simulink model "System_20220515"  (R2020b)
settings: Solver=ode4  StartTime=0.0  StopTime=inf  FixedStep=Ts  RelTol=1e-3  EnableMultiTasking=on
PreLoadFcn:
  | simulation_vars
PostLoadFcn:
  | simulation_vars
InitFcn:
  | simulation_vars
StartFcn:
  | simulation_vars
values from neighbouring files (symbols this model uses):
  ang_variance = 0.001*60    (= 0.06)    [simulation_vars.m]
  bus_va_seed = abs(round(1000*randn(73,1)))    [simulation_vars.m]
  bus_vm_seed = abs(round(1000*randn(73,1)))    [simulation_vars.m]
  event_time_end = event_time_start + 5/60    (= 10000.0833333)    [simulation_vars.m]
  event_time_start = 10000    [simulation_vars.m]
  line_iang0_seed = abs(round(1000*randn(104,1)))    [simulation_vars.m]
  line_iang1_seed = abs(round(1000*randn(104,1)))    [simulation_vars.m]
  line_imag0_seed = abs(round(1000*randn(104,1)))    [simulation_vars.m]
  line_imag1_seed = abs(round(1000*randn(104,1)))    [simulation_vars.m]
  mag_variance = 0.0005    [simulation_vars.m]
  spoof_lower_limit = -pi()/9    [simulation_vars.m]
  spoof_upper_limit = pi()/9    [simulation_vars.m]
  Ts = 0.001    [simulation_vars.m]
  xf_iang0_seed = abs(round(1000*randn(16,1)))    [simulation_vars.m]
  xf_iang1_seed = abs(round(1000*randn(16,1)))    [simulation_vars.m]
  xf_imag0_seed = abs(round(1000*randn(16,1)))    [simulation_vars.m]
  xf_imag1_seed = abs(round(1000*randn(16,1)))    [simulation_vars.m]
undefined symbols (not defined in the file or in its folder): en_spoofing_attack
libraries: rtlab x210, simulink x21, opal_lib x1, rtlab_phasor x1, rtio_spectracom x1
(part 3 of 4)

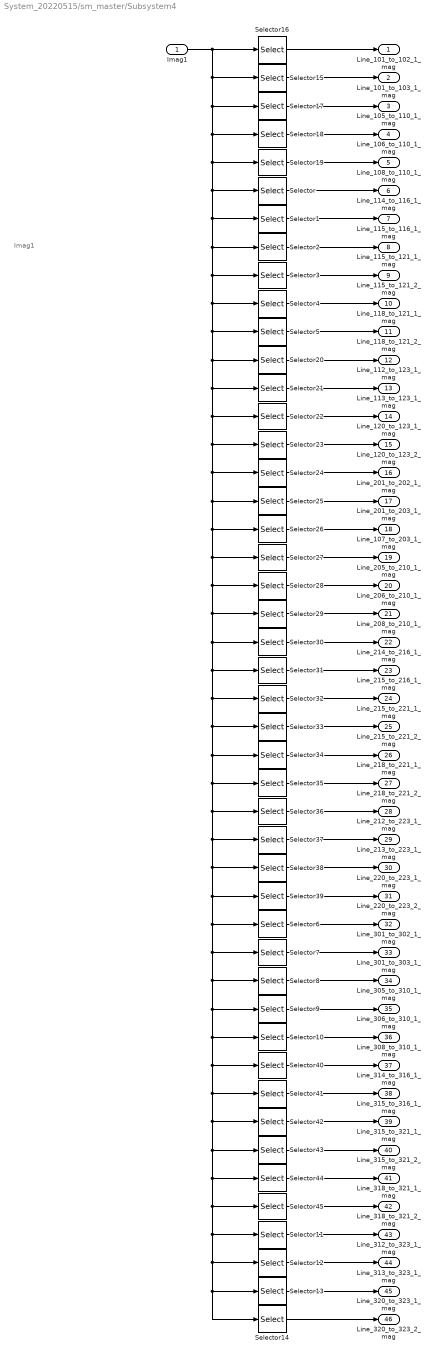
== system System_20220515/sm_master/Subsystem4 ==
  note: Imag1
  Imag1 : Inport
  Selector : Selector  InputPortWidth=104  IndexOptions=Index vector (dialog)  Indices=20  OutputSizes=1
  Selector1 : Selector  InputPortWidth=104  IndexOptions=Index vector (dialog)  Indices=21  OutputSizes=1
  Selector10 : Selector  InputPortWidth=104  IndexOptions=Index vector (dialog)  Indices=83  OutputSizes=1
  Selector11 : Selector  InputPortWidth=104  IndexOptions=Index vector (dialog)  Indices=87  OutputSizes=1
  Selector12 : Selector  InputPortWidth=104  IndexOptions=Index vector (dialog)  Indices=88  OutputSizes=1
  Selector13 : Selector  InputPortWidth=104  IndexOptions=Index vector (dialog)  Indices=102  OutputSizes=1
  Selector14 : Selector  InputPortWidth=104  IndexOptions=Index vector (dialog)  Indices=103  OutputSizes=1
  Selector15 : Selector  InputPortWidth=104  IndexOptions=Index vector (dialog)  Indices=2  OutputSizes=1
  Selector16 : Selector  InputPortWidth=104  IndexOptions=Index vector (dialog)  Indices=1  OutputSizes=1
  Selector17 : Selector  InputPortWidth=104  IndexOptions=Index vector (dialog)  Indices=8  OutputSizes=1
  Selector18 : Selector  InputPortWidth=104  IndexOptions=Index vector (dialog)  Indices=9  OutputSizes=1
  Selector19 : Selector  InputPortWidth=104  IndexOptions=Index vector (dialog)  Indices=13  OutputSizes=1
  Selector2 : Selector  InputPortWidth=104  IndexOptions=Index vector (dialog)  Indices=22  OutputSizes=1
  Selector20 : Selector  InputPortWidth=104  IndexOptions=Index vector (dialog)  Indices=17  OutputSizes=1
  Selector21 : Selector  InputPortWidth=104  IndexOptions=Index vector (dialog)  Indices=18  OutputSizes=1
  Selector22 : Selector  InputPortWidth=104  IndexOptions=Index vector (dialog)  Indices=33  OutputSizes=1
  Selector23 : Selector  InputPortWidth=104  IndexOptions=Index vector (dialog)  Indices=34  OutputSizes=1
  Selector24 : Selector  InputPortWidth=104  IndexOptions=Index vector (dialog)  Indices=38  OutputSizes=1
  Selector25 : Selector  InputPortWidth=104  IndexOptions=Index vector (dialog)  Indices=39  OutputSizes=1
  Selector26 : Selector  InputPortWidth=104  IndexOptions=Index vector (dialog)  Indices=11  OutputSizes=1
  Selector27 : Selector  InputPortWidth=104  IndexOptions=Index vector (dialog)  Indices=45  OutputSizes=1
  Selector28 : Selector  InputPortWidth=104  IndexOptions=Index vector (dialog)  Indices=46  OutputSizes=1
  Selector29 : Selector  InputPortWidth=104  IndexOptions=Index vector (dialog)  Indices=49  OutputSizes=1
  Selector3 : Selector  InputPortWidth=104  IndexOptions=Index vector (dialog)  Indices=23  OutputSizes=1
  Selector30 : Selector  InputPortWidth=104  IndexOptions=Index vector (dialog)  Indices=55  OutputSizes=1
  Selector31 : Selector  InputPortWidth=104  IndexOptions=Index vector (dialog)  Indices=56  OutputSizes=1
  Selector32 : Selector  InputPortWidth=104  IndexOptions=Index vector (dialog)  Indices=57  OutputSizes=1
  Selector33 : Selector  InputPortWidth=104  IndexOptions=Index vector (dialog)  Indices=58  OutputSizes=1
  Selector34 : Selector  InputPortWidth=104  IndexOptions=Index vector (dialog)  Indices=64  OutputSizes=1
  Selector35 : Selector  InputPortWidth=104  IndexOptions=Index vector (dialog)  Indices=65  OutputSizes=1
  Selector36 : Selector  InputPortWidth=104  IndexOptions=Index vector (dialog)  Indices=53  OutputSizes=1
  Selector37 : Selector  InputPortWidth=104  IndexOptions=Index vector (dialog)  Indices=54  OutputSizes=1
  Selector38 : Selector  InputPortWidth=104  IndexOptions=Index vector (dialog)  Indices=68  OutputSizes=1
  Selector39 : Selector  InputPortWidth=104  IndexOptions=Index vector (dialog)  Indices=69  OutputSizes=1
  Selector4 : Selector  InputPortWidth=104  IndexOptions=Index vector (dialog)  Indices=29  OutputSizes=1
  Selector40 : Selector  InputPortWidth=104  IndexOptions=Index vector (dialog)  Indices=89  OutputSizes=1
  Selector41 : Selector  InputPortWidth=104  IndexOptions=Index vector (dialog)  Indices=90  OutputSizes=1
  Selector42 : Selector  InputPortWidth=104  IndexOptions=Index vector (dialog)  Indices=91  OutputSizes=1
  Selector43 : Selector  InputPortWidth=104  IndexOptions=Index vector (dialog)  Indices=92  OutputSizes=1
  Selector44 : Selector  InputPortWidth=104  IndexOptions=Index vector (dialog)  Indices=98  OutputSizes=1
  Selector45 : Selector  InputPortWidth=104  IndexOptions=Index vector (dialog)  Indices=99  OutputSizes=1
  Selector5 : Selector  InputPortWidth=104  IndexOptions=Index vector (dialog)  Indices=30  OutputSizes=1
  Selector6 : Selector  InputPortWidth=104  IndexOptions=Index vector (dialog)  Indices=72  OutputSizes=1
  Selector7 : Selector  InputPortWidth=104  IndexOptions=Index vector (dialog)  Indices=73  OutputSizes=1
  Selector8 : Selector  InputPortWidth=104  IndexOptions=Index vector (dialog)  Indices=79  OutputSizes=1
  Selector9 : Selector  InputPortWidth=104  IndexOptions=Index vector (dialog)  Indices=80  OutputSizes=1
  Line_101_to_102_1_mag : Outport  VectorParamsAs1DForOutWhenUnconnected=off
  Line_101_to_103_1_mag : Outport  Port=2  VectorParamsAs1DForOutWhenUnconnected=off
  Line_105_to_110_1_mag : Outport  Port=3  VectorParamsAs1DForOutWhenUnconnected=off
  Line_106_to_110_1_mag : Outport  Port=4  VectorParamsAs1DForOutWhenUnconnected=off
  Line_108_to_110_1_mag : Outport  Port=5  VectorParamsAs1DForOutWhenUnconnected=off
  Line_114_to_116_1_mag : Outport  Port=6  VectorParamsAs1DForOutWhenUnconnected=off
  Line_115_to_116_1_mag : Outport  Port=7  VectorParamsAs1DForOutWhenUnconnected=off
  Line_115_to_121_1_mag : Outport  Port=8  VectorParamsAs1DForOutWhenUnconnected=off
  Line_115_to_121_2_mag : Outport  Port=9  VectorParamsAs1DForOutWhenUnconnected=off
  Line_118_to_121_1_mag : Outport  Port=10  VectorParamsAs1DForOutWhenUnconnected=off
  Line_118_to_121_2_mag : Outport  Port=11  VectorParamsAs1DForOutWhenUnconnected=off
  Line_112_to_123_1_mag : Outport  Port=12  VectorParamsAs1DForOutWhenUnconnected=off
  Line_113_to_123_1_mag : Outport  Port=13  VectorParamsAs1DForOutWhenUnconnected=off
  Line_120_to_123_1_mag : Outport  Port=14  VectorParamsAs1DForOutWhenUnconnected=off
  Line_120_to_123_2_mag : Outport  Port=15  VectorParamsAs1DForOutWhenUnconnected=off
  Line_201_to_202_1_mag : Outport  Port=16  VectorParamsAs1DForOutWhenUnconnected=off
  Line_201_to_203_1_mag : Outport  Port=17  VectorParamsAs1DForOutWhenUnconnected=off
  Line_107_to_203_1_mag : Outport  Port=18  VectorParamsAs1DForOutWhenUnconnected=off
  Line_205_to_210_1_mag : Outport  Port=19  VectorParamsAs1DForOutWhenUnconnected=off
  Line_206_to_210_1_mag : Outport  Port=20  VectorParamsAs1DForOutWhenUnconnected=off
  Line_208_to_210_1_mag : Outport  Port=21  VectorParamsAs1DForOutWhenUnconnected=off
  Line_214_to_216_1_mag : Outport  Port=22  VectorParamsAs1DForOutWhenUnconnected=off
  Line_215_to_216_1_mag : Outport  Port=23  VectorParamsAs1DForOutWhenUnconnected=off
  Line_215_to_221_1_mag : Outport  Port=24  VectorParamsAs1DForOutWhenUnconnected=off
  Line_215_to_221_2_mag : Outport  Port=25  VectorParamsAs1DForOutWhenUnconnected=off
  Line_218_to_221_1_mag : Outport  Port=26  VectorParamsAs1DForOutWhenUnconnected=off
  Line_218_to_221_2_mag : Outport  Port=27  VectorParamsAs1DForOutWhenUnconnected=off
  Line_212_to_223_1_mag : Outport  Port=28  VectorParamsAs1DForOutWhenUnconnected=off
  Line_213_to_223_1_mag : Outport  Port=29  VectorParamsAs1DForOutWhenUnconnected=off
  Line_220_to_223_1_mag : Outport  Port=30  VectorParamsAs1DForOutWhenUnconnected=off
  Line_220_to_223_2_mag : Outport  Port=31  VectorParamsAs1DForOutWhenUnconnected=off
  Line_301_to_302_1_mag : Outport  Port=32  VectorParamsAs1DForOutWhenUnconnected=off
  Line_301_to_303_1_mag : Outport  Port=33  VectorParamsAs1DForOutWhenUnconnected=off
  Line_305_to_310_1_mag : Outport  Port=34  VectorParamsAs1DForOutWhenUnconnected=off
  Line_306_to_310_1_mag : Outport  Port=35  VectorParamsAs1DForOutWhenUnconnected=off
  Line_308_to_310_1_mag : Outport  Port=36  VectorParamsAs1DForOutWhenUnconnected=off
  Line_314_to_316_1_mag : Outport  Port=37  VectorParamsAs1DForOutWhenUnconnected=off
  Line_315_to_316_1_mag : Outport  Port=38  VectorParamsAs1DForOutWhenUnconnected=off
  Line_315_to_321_1_mag : Outport  Port=39  VectorParamsAs1DForOutWhenUnconnected=off
  Line_315_to_321_2_mag : Outport  Port=40  VectorParamsAs1DForOutWhenUnconnected=off
  Line_318_to_321_1_mag : Outport  Port=41  VectorParamsAs1DForOutWhenUnconnected=off
  Line_318_to_321_2_mag : Outport  Port=42  VectorParamsAs1DForOutWhenUnconnected=off
  Line_312_to_323_1_mag : Outport  Port=43  VectorParamsAs1DForOutWhenUnconnected=off
  Line_313_to_323_1_mag : Outport  Port=44  VectorParamsAs1DForOutWhenUnconnected=off
  Line_320_to_323_1_mag : Outport  Port=45  VectorParamsAs1DForOutWhenUnconnected=off
  Line_320_to_323_2_mag : Outport  Port=46  VectorParamsAs1DForOutWhenUnconnected=off
  wires:
  Selector/1 -> Line_114_to_116_1_mag/1
  Selector1/1 -> Line_115_to_116_1_mag/1
  Selector2/1 -> Line_115_to_121_1_mag/1
  Selector3/1 -> Line_115_to_121_2_mag/1
  Selector4/1 -> Line_118_to_121_1_mag/1
  Selector5/1 -> Line_118_to_121_2_mag/1
  Selector6/1 -> Line_301_to_302_1_mag/1
  Selector7/1 -> Line_301_to_303_1_mag/1
  Selector8/1 -> Line_305_to_310_1_mag/1
  Selector9/1 -> Line_306_to_310_1_mag/1
  Selector10/1 -> Line_308_to_310_1_mag/1
  Selector11/1 -> Line_312_to_323_1_mag/1
  Selector12/1 -> Line_313_to_323_1_mag/1
  Selector13/1 -> Line_320_to_323_1_mag/1
  Selector14/1 -> Line_320_to_323_2_mag/1
  Imag1/1 -> Selector17/1, Selector18/1, Selector19/1, Selector4/1, Selector5/1, Selector20/1, Selector21/1, Selector22/1, Selector23/1, Selector24/1, Selector25/1, Selector26/1, Selector27/1, Selector28/1, Selector29/1, Selector30/1, Selector31/1, Selector32/1, Selector33/1, Selector34/1, Selector35/1, Selector36/1, Selector37/1, Selector38/1, Selector39/1, Selector8/1, Selector9/1, Selector10/1, Selector40/1, Selector41/1, Selector42/1, Selector43/1, Selector44/1, Selector45/1, Selector12/1, Selector13/1, Selector14/1, Selector11/1, Selector7/1, Selector6/1, Selector3/1, Selector2/1, Selector1/1, Selector/1, Selector15/1, Selector16/1
  Selector16/1 -> Line_101_to_102_1_mag/1
  Selector15/1 -> Line_101_to_103_1_mag/1
  Selector17/1 -> Line_105_to_110_1_mag/1
  Selector18/1 -> Line_106_to_110_1_mag/1
  Selector19/1 -> Line_108_to_110_1_mag/1
  Selector20/1 -> Line_112_to_123_1_mag/1
  Selector21/1 -> Line_113_to_123_1_mag/1
  Selector22/1 -> Line_120_to_123_1_mag/1
  Selector23/1 -> Line_120_to_123_2_mag/1
  Selector24/1 -> Line_201_to_202_1_mag/1
  Selector25/1 -> Line_201_to_203_1_mag/1
  Selector26/1 -> Line_107_to_203_1_mag/1
  Selector27/1 -> Line_205_to_210_1_mag/1
  Selector28/1 -> Line_206_to_210_1_mag/1
  Selector29/1 -> Line_208_to_210_1_mag/1
  Selector30/1 -> Line_214_to_216_1_mag/1
  Selector31/1 -> Line_215_to_216_1_mag/1
  Selector32/1 -> Line_215_to_221_1_mag/1
  Selector33/1 -> Line_215_to_221_2_mag/1
  Selector34/1 -> Line_218_to_221_1_mag/1
  Selector35/1 -> Line_218_to_221_2_mag/1
  Selector36/1 -> Line_212_to_223_1_mag/1
  Selector37/1 -> Line_213_to_223_1_mag/1
  Selector38/1 -> Line_220_to_223_1_mag/1
  Selector39/1 -> Line_220_to_223_2_mag/1
  Selector40/1 -> Line_314_to_316_1_mag/1
  Selector41/1 -> Line_315_to_316_1_mag/1
  Selector42/1 -> Line_315_to_321_1_mag/1
  Selector43/1 -> Line_315_to_321_2_mag/1
  Selector44/1 -> Line_318_to_321_1_mag/1
  Selector45/1 -> Line_318_to_321_2_mag/1

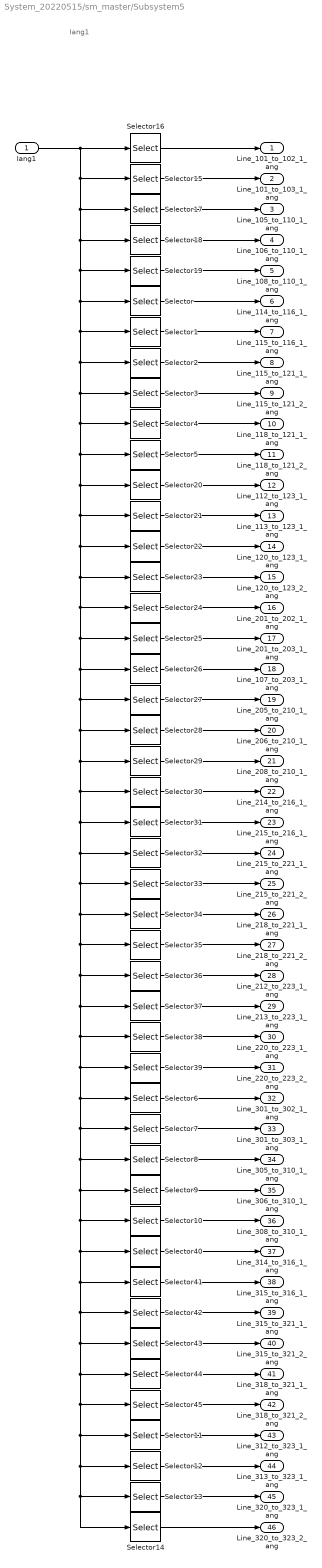
== system System_20220515/sm_master/Subsystem5 ==
  note: Iang1
  Iang1 : Inport
  Selector : Selector  InputPortWidth=104  IndexOptions=Index vector (dialog)  Indices=20  OutputSizes=1
  Selector1 : Selector  InputPortWidth=104  IndexOptions=Index vector (dialog)  Indices=21  OutputSizes=1
  Selector10 : Selector  InputPortWidth=104  IndexOptions=Index vector (dialog)  Indices=83  OutputSizes=1
  Selector11 : Selector  InputPortWidth=104  IndexOptions=Index vector (dialog)  Indices=87  OutputSizes=1
  Selector12 : Selector  InputPortWidth=104  IndexOptions=Index vector (dialog)  Indices=88  OutputSizes=1
  Selector13 : Selector  InputPortWidth=104  IndexOptions=Index vector (dialog)  Indices=102  OutputSizes=1
  Selector14 : Selector  InputPortWidth=104  IndexOptions=Index vector (dialog)  Indices=103  OutputSizes=1
  Selector15 : Selector  InputPortWidth=104  IndexOptions=Index vector (dialog)  Indices=2  OutputSizes=1
  Selector16 : Selector  InputPortWidth=104  IndexOptions=Index vector (dialog)  Indices=1  OutputSizes=1
  Selector17 : Selector  InputPortWidth=104  IndexOptions=Index vector (dialog)  Indices=8  OutputSizes=1
  Selector18 : Selector  InputPortWidth=104  IndexOptions=Index vector (dialog)  Indices=9  OutputSizes=1
  Selector19 : Selector  InputPortWidth=104  IndexOptions=Index vector (dialog)  Indices=13  OutputSizes=1
  Selector2 : Selector  InputPortWidth=104  IndexOptions=Index vector (dialog)  Indices=22  OutputSizes=1
  Selector20 : Selector  InputPortWidth=104  IndexOptions=Index vector (dialog)  Indices=17  OutputSizes=1
  Selector21 : Selector  InputPortWidth=104  IndexOptions=Index vector (dialog)  Indices=18  OutputSizes=1
  Selector22 : Selector  InputPortWidth=104  IndexOptions=Index vector (dialog)  Indices=33  OutputSizes=1
  Selector23 : Selector  InputPortWidth=104  IndexOptions=Index vector (dialog)  Indices=34  OutputSizes=1
  Selector24 : Selector  InputPortWidth=104  IndexOptions=Index vector (dialog)  Indices=38  OutputSizes=1
  Selector25 : Selector  InputPortWidth=104  IndexOptions=Index vector (dialog)  Indices=39  OutputSizes=1
  Selector26 : Selector  InputPortWidth=104  IndexOptions=Index vector (dialog)  Indices=11  OutputSizes=1
  Selector27 : Selector  InputPortWidth=104  IndexOptions=Index vector (dialog)  Indices=45  OutputSizes=1
  Selector28 : Selector  InputPortWidth=104  IndexOptions=Index vector (dialog)  Indices=46  OutputSizes=1
  Selector29 : Selector  InputPortWidth=104  IndexOptions=Index vector (dialog)  Indices=49  OutputSizes=1
  Selector3 : Selector  InputPortWidth=104  IndexOptions=Index vector (dialog)  Indices=23  OutputSizes=1
  Selector30 : Selector  InputPortWidth=104  IndexOptions=Index vector (dialog)  Indices=55  OutputSizes=1
  Selector31 : Selector  InputPortWidth=104  IndexOptions=Index vector (dialog)  Indices=56  OutputSizes=1
  Selector32 : Selector  InputPortWidth=104  IndexOptions=Index vector (dialog)  Indices=57  OutputSizes=1
  Selector33 : Selector  InputPortWidth=104  IndexOptions=Index vector (dialog)  Indices=58  OutputSizes=1
  Selector34 : Selector  InputPortWidth=104  IndexOptions=Index vector (dialog)  Indices=64  OutputSizes=1
  Selector35 : Selector  InputPortWidth=104  IndexOptions=Index vector (dialog)  Indices=65  OutputSizes=1
  Selector36 : Selector  InputPortWidth=104  IndexOptions=Index vector (dialog)  Indices=53  OutputSizes=1
  Selector37 : Selector  InputPortWidth=104  IndexOptions=Index vector (dialog)  Indices=54  OutputSizes=1
  Selector38 : Selector  InputPortWidth=104  IndexOptions=Index vector (dialog)  Indices=68  OutputSizes=1
  Selector39 : Selector  InputPortWidth=104  IndexOptions=Index vector (dialog)  Indices=69  OutputSizes=1
  Selector4 : Selector  InputPortWidth=104  IndexOptions=Index vector (dialog)  Indices=29  OutputSizes=1
  Selector40 : Selector  InputPortWidth=104  IndexOptions=Index vector (dialog)  Indices=89  OutputSizes=1
  Selector41 : Selector  InputPortWidth=104  IndexOptions=Index vector (dialog)  Indices=90  OutputSizes=1
  Selector42 : Selector  InputPortWidth=104  IndexOptions=Index vector (dialog)  Indices=91  OutputSizes=1
  Selector43 : Selector  InputPortWidth=104  IndexOptions=Index vector (dialog)  Indices=92  OutputSizes=1
  Selector44 : Selector  InputPortWidth=104  IndexOptions=Index vector (dialog)  Indices=98  OutputSizes=1
  Selector45 : Selector  InputPortWidth=104  IndexOptions=Index vector (dialog)  Indices=99  OutputSizes=1
  Selector5 : Selector  InputPortWidth=104  IndexOptions=Index vector (dialog)  Indices=30  OutputSizes=1
  Selector6 : Selector  InputPortWidth=104  IndexOptions=Index vector (dialog)  Indices=72  OutputSizes=1
  Selector7 : Selector  InputPortWidth=104  IndexOptions=Index vector (dialog)  Indices=73  OutputSizes=1
  Selector8 : Selector  InputPortWidth=104  IndexOptions=Index vector (dialog)  Indices=79  OutputSizes=1
  Selector9 : Selector  InputPortWidth=104  IndexOptions=Index vector (dialog)  Indices=80  OutputSizes=1
  Line_101_to_102_1_ang : Outport  VectorParamsAs1DForOutWhenUnconnected=off
  Line_101_to_103_1_ang : Outport  Port=2  VectorParamsAs1DForOutWhenUnconnected=off
  Line_105_to_110_1_ang : Outport  Port=3  VectorParamsAs1DForOutWhenUnconnected=off
  Line_106_to_110_1_ang : Outport  Port=4  VectorParamsAs1DForOutWhenUnconnected=off
  Line_108_to_110_1_ang : Outport  Port=5  VectorParamsAs1DForOutWhenUnconnected=off
  Line_114_to_116_1_ang : Outport  Port=6  VectorParamsAs1DForOutWhenUnconnected=off
  Line_115_to_116_1_ang : Outport  Port=7  VectorParamsAs1DForOutWhenUnconnected=off
  Line_115_to_121_1_ang : Outport  Port=8  VectorParamsAs1DForOutWhenUnconnected=off
  Line_115_to_121_2_ang : Outport  Port=9  VectorParamsAs1DForOutWhenUnconnected=off
  Line_118_to_121_1_ang : Outport  Port=10  VectorParamsAs1DForOutWhenUnconnected=off
  Line_118_to_121_2_ang : Outport  Port=11  VectorParamsAs1DForOutWhenUnconnected=off
  Line_112_to_123_1_ang : Outport  Port=12  VectorParamsAs1DForOutWhenUnconnected=off
  Line_113_to_123_1_ang : Outport  Port=13  VectorParamsAs1DForOutWhenUnconnected=off
  Line_120_to_123_1_ang : Outport  Port=14  VectorParamsAs1DForOutWhenUnconnected=off
  Line_120_to_123_2_ang : Outport  Port=15  VectorParamsAs1DForOutWhenUnconnected=off
  Line_201_to_202_1_ang : Outport  Port=16  VectorParamsAs1DForOutWhenUnconnected=off
  Line_201_to_203_1_ang : Outport  Port=17  VectorParamsAs1DForOutWhenUnconnected=off
  Line_107_to_203_1_ang : Outport  Port=18  VectorParamsAs1DForOutWhenUnconnected=off
  Line_205_to_210_1_ang : Outport  Port=19  VectorParamsAs1DForOutWhenUnconnected=off
  Line_206_to_210_1_ang : Outport  Port=20  VectorParamsAs1DForOutWhenUnconnected=off
  Line_208_to_210_1_ang : Outport  Port=21  VectorParamsAs1DForOutWhenUnconnected=off
  Line_214_to_216_1_ang : Outport  Port=22  VectorParamsAs1DForOutWhenUnconnected=off
  Line_215_to_216_1_ang : Outport  Port=23  VectorParamsAs1DForOutWhenUnconnected=off
  Line_215_to_221_1_ang : Outport  Port=24  VectorParamsAs1DForOutWhenUnconnected=off
  Line_215_to_221_2_ang : Outport  Port=25  VectorParamsAs1DForOutWhenUnconnected=off
  Line_218_to_221_1_ang : Outport  Port=26  VectorParamsAs1DForOutWhenUnconnected=off
  Line_218_to_221_2_ang : Outport  Port=27  VectorParamsAs1DForOutWhenUnconnected=off
  Line_212_to_223_1_ang : Outport  Port=28  VectorParamsAs1DForOutWhenUnconnected=off
  Line_213_to_223_1_ang : Outport  Port=29  VectorParamsAs1DForOutWhenUnconnected=off
  Line_220_to_223_1_ang : Outport  Port=30  VectorParamsAs1DForOutWhenUnconnected=off
  Line_220_to_223_2_ang : Outport  Port=31  VectorParamsAs1DForOutWhenUnconnected=off
  Line_301_to_302_1_ang : Outport  Port=32  VectorParamsAs1DForOutWhenUnconnected=off
  Line_301_to_303_1_ang : Outport  Port=33  VectorParamsAs1DForOutWhenUnconnected=off
  Line_305_to_310_1_ang : Outport  Port=34  VectorParamsAs1DForOutWhenUnconnected=off
  Line_306_to_310_1_ang : Outport  Port=35  VectorParamsAs1DForOutWhenUnconnected=off
  Line_308_to_310_1_ang : Outport  Port=36  VectorParamsAs1DForOutWhenUnconnected=off
  Line_314_to_316_1_ang : Outport  Port=37  VectorParamsAs1DForOutWhenUnconnected=off
  Line_315_to_316_1_ang : Outport  Port=38  VectorParamsAs1DForOutWhenUnconnected=off
  Line_315_to_321_1_ang : Outport  Port=39  VectorParamsAs1DForOutWhenUnconnected=off
  Line_315_to_321_2_ang : Outport  Port=40  VectorParamsAs1DForOutWhenUnconnected=off
  Line_318_to_321_1_ang : Outport  Port=41  VectorParamsAs1DForOutWhenUnconnected=off
  Line_318_to_321_2_ang : Outport  Port=42  VectorParamsAs1DForOutWhenUnconnected=off
  Line_312_to_323_1_ang : Outport  Port=43  VectorParamsAs1DForOutWhenUnconnected=off
  Line_313_to_323_1_ang : Outport  Port=44  VectorParamsAs1DForOutWhenUnconnected=off
  Line_320_to_323_1_ang : Outport  Port=45  VectorParamsAs1DForOutWhenUnconnected=off
  Line_320_to_323_2_ang : Outport  Port=46  VectorParamsAs1DForOutWhenUnconnected=off
  wires:
  Selector44/1 -> Line_318_to_321_1_ang/1
  Selector25/1 -> Line_201_to_203_1_ang/1
  Selector28/1 -> Line_206_to_210_1_ang/1
  Selector45/1 -> Line_318_to_321_2_ang/1
  Selector38/1 -> Line_220_to_223_1_ang/1
  Selector32/1 -> Line_215_to_221_1_ang/1
  Selector37/1 -> Line_213_to_223_1_ang/1
  Selector26/1 -> Line_107_to_203_1_ang/1
  Selector18/1 -> Line_106_to_110_1_ang/1
  Selector36/1 -> Line_212_to_223_1_ang/1
  Selector19/1 -> Line_108_to_110_1_ang/1
  Selector23/1 -> Line_120_to_123_2_ang/1
  Selector31/1 -> Line_215_to_216_1_ang/1
  Selector33/1 -> Line_215_to_221_2_ang/1
  Selector41/1 -> Line_315_to_316_1_ang/1
  Selector35/1 -> Line_218_to_221_2_ang/1
  Selector17/1 -> Line_105_to_110_1_ang/1
  Selector43/1 -> Line_315_to_321_2_ang/1
  Selector20/1 -> Line_112_to_123_1_ang/1
  Selector9/1 -> Line_306_to_310_1_ang/1
  Selector/1 -> Line_114_to_116_1_ang/1
  Iang1/1 -> Selector17/1, Selector18/1, Selector19/1, Selector4/1, Selector5/1, Selector20/1, Selector21/1, Selector22/1, Selector23/1, Selector24/1, Selector25/1, Selector26/1, Selector27/1, Selector28/1, Selector29/1, Selector30/1, Selector31/1, Selector32/1, Selector33/1, Selector34/1, Selector35/1, Selector36/1, Selector37/1, Selector38/1, Selector39/1, Selector8/1, Selector9/1, Selector10/1, Selector40/1, Selector41/1, Selector42/1, Selector43/1, Selector44/1, Selector45/1, Selector12/1, Selector13/1, Selector14/1, Selector11/1, Selector7/1, Selector6/1, Selector3/1, Selector2/1, Selector1/1, Selector/1, Selector15/1, Selector16/1
  Selector14/1 -> Line_320_to_323_2_ang/1
  Selector1/1 -> Line_115_to_116_1_ang/1
  Selector13/1 -> Line_320_to_323_1_ang/1
  Selector12/1 -> Line_313_to_323_1_ang/1
  Selector4/1 -> Line_118_to_121_1_ang/1
  Selector7/1 -> Line_301_to_303_1_ang/1
  Selector2/1 -> Line_115_to_121_1_ang/1
  Selector6/1 -> Line_301_to_302_1_ang/1
  Selector42/1 -> Line_315_to_321_1_ang/1
  Selector21/1 -> Line_113_to_123_1_ang/1
  Selector22/1 -> Line_120_to_123_1_ang/1
  Selector15/1 -> Line_101_to_103_1_ang/1
  Selector16/1 -> Line_101_to_102_1_ang/1
  Selector27/1 -> Line_205_to_210_1_ang/1
  Selector30/1 -> Line_214_to_216_1_ang/1
  Selector3/1 -> Line_115_to_121_2_ang/1
  Selector8/1 -> Line_305_to_310_1_ang/1
  Selector39/1 -> Line_220_to_223_2_ang/1
  Selector40/1 -> Line_314_to_316_1_ang/1
  Selector29/1 -> Line_208_to_210_1_ang/1
  Selector11/1 -> Line_312_to_323_1_ang/1
  Selector34/1 -> Line_218_to_221_1_ang/1
  Selector24/1 -> Line_201_to_202_1_ang/1
  Selector10/1 -> Line_308_to_310_1_ang/1
  Selector5/1 -> Line_118_to_121_2_ang/1

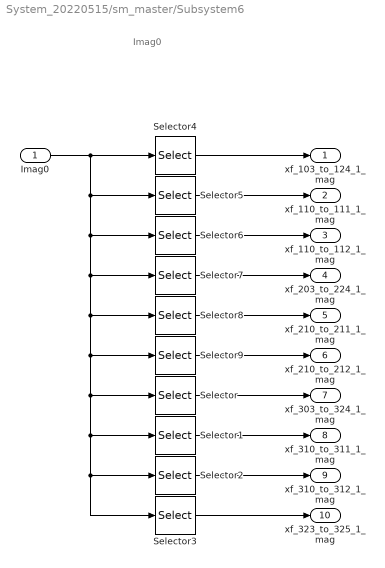
== system System_20220515/sm_master/Subsystem6 ==
  note: Imag0
  Imag0 : Inport
  Selector : Selector  InputPortWidth=16  IndexOptions=Index vector (dialog)  Indices=11  OutputSizes=1
  Selector1 : Selector  InputPortWidth=16  IndexOptions=Index vector (dialog)  Indices=14  OutputSizes=1
  Selector2 : Selector  InputPortWidth=16  IndexOptions=Index vector (dialog)  Indices=15  OutputSizes=1
  Selector3 : Selector  InputPortWidth=16  IndexOptions=Index vector (dialog)  Indices=16  OutputSizes=1
  Selector4 : Selector  InputPortWidth=16  IndexOptions=Index vector (dialog)  Indices=1  OutputSizes=1
  Selector5 : Selector  InputPortWidth=16  IndexOptions=Index vector (dialog)  Indices=4  OutputSizes=1
  Selector6 : Selector  InputPortWidth=16  IndexOptions=Index vector (dialog)  Indices=5  OutputSizes=1
  Selector7 : Selector  InputPortWidth=16  IndexOptions=Index vector (dialog)  Indices=6  OutputSizes=1
  Selector8 : Selector  InputPortWidth=16  IndexOptions=Index vector (dialog)  Indices=9  OutputSizes=1
  Selector9 : Selector  InputPortWidth=16  IndexOptions=Index vector (dialog)  Indices=10  OutputSizes=1
  xf_103_to_124_1_mag : Outport  VectorParamsAs1DForOutWhenUnconnected=off
  xf_110_to_111_1_mag : Outport  Port=2  VectorParamsAs1DForOutWhenUnconnected=off
  xf_110_to_112_1_mag : Outport  Port=3  VectorParamsAs1DForOutWhenUnconnected=off
  xf_203_to_224_1_mag : Outport  Port=4  VectorParamsAs1DForOutWhenUnconnected=off
  xf_210_to_211_1_mag : Outport  Port=5  VectorParamsAs1DForOutWhenUnconnected=off
  xf_210_to_212_1_mag : Outport  Port=6  VectorParamsAs1DForOutWhenUnconnected=off
  xf_303_to_324_1_mag : Outport  Port=7  VectorParamsAs1DForOutWhenUnconnected=off
  xf_310_to_311_1_mag : Outport  Port=8  VectorParamsAs1DForOutWhenUnconnected=off
  xf_310_to_312_1_mag : Outport  Port=9  VectorParamsAs1DForOutWhenUnconnected=off
  xf_323_to_325_1_mag : Outport  Port=10  VectorParamsAs1DForOutWhenUnconnected=off
  wires:
  Selector/1 -> xf_303_to_324_1_mag/1
  Selector1/1 -> xf_310_to_311_1_mag/1
  Selector2/1 -> xf_310_to_312_1_mag/1
  Imag0/1 -> Selector4/1, Selector5/1, Selector6/1, Selector7/1, Selector3/1, Selector2/1, Selector1/1, Selector/1, Selector9/1, Selector8/1
  Selector3/1 -> xf_323_to_325_1_mag/1
  Selector4/1 -> xf_103_to_124_1_mag/1
  Selector5/1 -> xf_110_to_111_1_mag/1
  Selector6/1 -> xf_110_to_112_1_mag/1
  Selector7/1 -> xf_203_to_224_1_mag/1
  Selector8/1 -> xf_210_to_211_1_mag/1
  Selector9/1 -> xf_210_to_212_1_mag/1

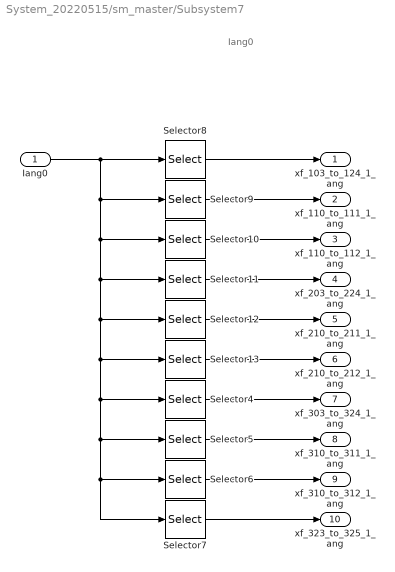
== system System_20220515/sm_master/Subsystem7 ==
  note: Iang0
  Iang0 : Inport
  Selector10 : Selector  InputPortWidth=16  IndexOptions=Index vector (dialog)  Indices=5  OutputSizes=1
  Selector11 : Selector  InputPortWidth=16  IndexOptions=Index vector (dialog)  Indices=6  OutputSizes=1
  Selector12 : Selector  InputPortWidth=16  IndexOptions=Index vector (dialog)  Indices=9  OutputSizes=1
  Selector13 : Selector  InputPortWidth=16  IndexOptions=Index vector (dialog)  Indices=10  OutputSizes=1
  Selector4 : Selector  InputPortWidth=16  IndexOptions=Index vector (dialog)  Indices=11  OutputSizes=1
  Selector5 : Selector  InputPortWidth=16  IndexOptions=Index vector (dialog)  Indices=14  OutputSizes=1
  Selector6 : Selector  InputPortWidth=16  IndexOptions=Index vector (dialog)  Indices=15  OutputSizes=1
  Selector7 : Selector  InputPortWidth=16  IndexOptions=Index vector (dialog)  Indices=16  OutputSizes=1
  Selector8 : Selector  InputPortWidth=16  IndexOptions=Index vector (dialog)  Indices=1  OutputSizes=1
  Selector9 : Selector  InputPortWidth=16  IndexOptions=Index vector (dialog)  Indices=4  OutputSizes=1
  xf_103_to_124_1_ang : Outport  VectorParamsAs1DForOutWhenUnconnected=off
  xf_110_to_111_1_ang : Outport  Port=2  VectorParamsAs1DForOutWhenUnconnected=off
  xf_110_to_112_1_ang : Outport  Port=3  VectorParamsAs1DForOutWhenUnconnected=off
  xf_203_to_224_1_ang : Outport  Port=4  VectorParamsAs1DForOutWhenUnconnected=off
  xf_210_to_211_1_ang : Outport  Port=5  VectorParamsAs1DForOutWhenUnconnected=off
  xf_210_to_212_1_ang : Outport  Port=6  VectorParamsAs1DForOutWhenUnconnected=off
  xf_303_to_324_1_ang : Outport  Port=7  VectorParamsAs1DForOutWhenUnconnected=off
  xf_310_to_311_1_ang : Outport  Port=8  VectorParamsAs1DForOutWhenUnconnected=off
  xf_310_to_312_1_ang : Outport  Port=9  VectorParamsAs1DForOutWhenUnconnected=off
  xf_323_to_325_1_ang : Outport  Port=10  VectorParamsAs1DForOutWhenUnconnected=off
  wires:
  Selector13/1 -> xf_210_to_212_1_ang/1
  Selector10/1 -> xf_110_to_112_1_ang/1
  Selector12/1 -> xf_210_to_211_1_ang/1
  Selector11/1 -> xf_203_to_224_1_ang/1
  Selector4/1 -> xf_303_to_324_1_ang/1
  Iang0/1 -> Selector8/1, Selector9/1, Selector10/1, Selector11/1, Selector7/1, Selector6/1, Selector5/1, Selector4/1, Selector13/1, Selector12/1
  Selector9/1 -> xf_110_to_111_1_ang/1
  Selector7/1 -> xf_323_to_325_1_ang/1
  Selector6/1 -> xf_310_to_312_1_ang/1
  Selector5/1 -> xf_310_to_311_1_ang/1
  Selector8/1 -> xf_103_to_124_1_ang/1

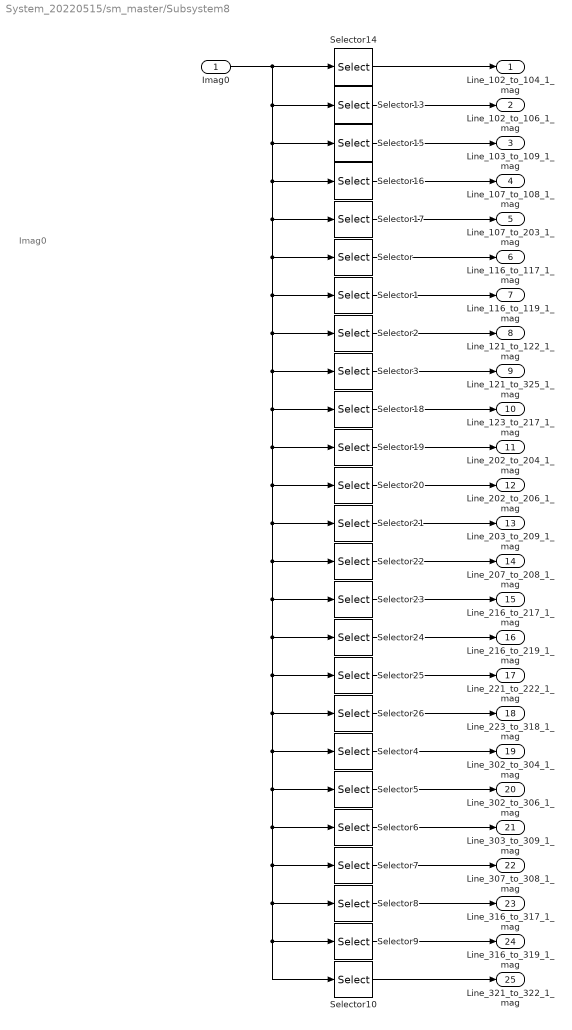
== system System_20220515/sm_master/Subsystem8 ==
  note: Imag0
  Imag0 : Inport
  Selector : Selector  InputPortWidth=104  IndexOptions=Index vector (dialog)  Indices=25  OutputSizes=1
  Selector1 : Selector  InputPortWidth=104  IndexOptions=Index vector (dialog)  Indices=26  OutputSizes=1
  Selector10 : Selector  InputPortWidth=104  IndexOptions=Index vector (dialog)  Indices=104  OutputSizes=1
  Selector13 : Selector  InputPortWidth=104  IndexOptions=Index vector (dialog)  Indices=5  OutputSizes=1
  Selector14 : Selector  InputPortWidth=104  IndexOptions=Index vector (dialog)  Indices=4  OutputSizes=1
  Selector15 : Selector  InputPortWidth=104  IndexOptions=Index vector (dialog)  Indices=6  OutputSizes=1
  Selector16 : Selector  InputPortWidth=104  IndexOptions=Index vector (dialog)  Indices=10  OutputSizes=1
  Selector17 : Selector  InputPortWidth=104  IndexOptions=Index vector (dialog)  Indices=11  OutputSizes=1
  Selector18 : Selector  InputPortWidth=104  IndexOptions=Index vector (dialog)  Indices=37  OutputSizes=1
  Selector19 : Selector  InputPortWidth=104  IndexOptions=Index vector (dialog)  Indices=41  OutputSizes=1
  Selector2 : Selector  InputPortWidth=104  IndexOptions=Index vector (dialog)  Indices=35  OutputSizes=1
  Selector20 : Selector  InputPortWidth=104  IndexOptions=Index vector (dialog)  Indices=42  OutputSizes=1
  Selector21 : Selector  InputPortWidth=104  IndexOptions=Index vector (dialog)  Indices=43  OutputSizes=1
  Selector22 : Selector  InputPortWidth=104  IndexOptions=Index vector (dialog)  Indices=47  OutputSizes=1
  Selector23 : Selector  InputPortWidth=104  IndexOptions=Index vector (dialog)  Indices=60  OutputSizes=1
  Selector24 : Selector  InputPortWidth=104  IndexOptions=Index vector (dialog)  Indices=61  OutputSizes=1
  Selector25 : Selector  InputPortWidth=104  IndexOptions=Index vector (dialog)  Indices=70  OutputSizes=1
  Selector26 : Selector  InputPortWidth=104  IndexOptions=Index vector (dialog)  Indices=71  OutputSizes=1
  Selector3 : Selector  InputPortWidth=104  IndexOptions=Index vector (dialog)  Indices=36  OutputSizes=1
  Selector4 : Selector  InputPortWidth=104  IndexOptions=Index vector (dialog)  Indices=75  OutputSizes=1
  Selector5 : Selector  InputPortWidth=104  IndexOptions=Index vector (dialog)  Indices=76  OutputSizes=1
  Selector6 : Selector  InputPortWidth=104  IndexOptions=Index vector (dialog)  Indices=77  OutputSizes=1
  Selector7 : Selector  InputPortWidth=104  IndexOptions=Index vector (dialog)  Indices=81  OutputSizes=1
  Selector8 : Selector  InputPortWidth=104  IndexOptions=Index vector (dialog)  Indices=94  OutputSizes=1
  Selector9 : Selector  InputPortWidth=104  IndexOptions=Index vector (dialog)  Indices=95  OutputSizes=1
  Line_102_to_104_1_mag : Outport  VectorParamsAs1DForOutWhenUnconnected=off
  Line_102_to_106_1_mag : Outport  Port=2  VectorParamsAs1DForOutWhenUnconnected=off
  Line_103_to_109_1_mag : Outport  Port=3  VectorParamsAs1DForOutWhenUnconnected=off
  Line_107_to_108_1_mag : Outport  Port=4  VectorParamsAs1DForOutWhenUnconnected=off
  Line_107_to_203_1_mag : Outport  Port=5  VectorParamsAs1DForOutWhenUnconnected=off
  Line_116_to_117_1_mag : Outport  Port=6  VectorParamsAs1DForOutWhenUnconnected=off
  Line_116_to_119_1_mag : Outport  Port=7  VectorParamsAs1DForOutWhenUnconnected=off
  Line_121_to_122_1_mag : Outport  Port=8  VectorParamsAs1DForOutWhenUnconnected=off
  Line_121_to_325_1_mag : Outport  Port=9  VectorParamsAs1DForOutWhenUnconnected=off
  Line_123_to_217_1_mag : Outport  Port=10  VectorParamsAs1DForOutWhenUnconnected=off
  Line_202_to_204_1_mag : Outport  Port=11  VectorParamsAs1DForOutWhenUnconnected=off
  Line_202_to_206_1_mag : Outport  Port=12  VectorParamsAs1DForOutWhenUnconnected=off
  Line_203_to_209_1_mag : Outport  Port=13  VectorParamsAs1DForOutWhenUnconnected=off
  Line_207_to_208_1_mag : Outport  Port=14  VectorParamsAs1DForOutWhenUnconnected=off
  Line_216_to_217_1_mag : Outport  Port=15  VectorParamsAs1DForOutWhenUnconnected=off
  Line_216_to_219_1_mag : Outport  Port=16  VectorParamsAs1DForOutWhenUnconnected=off
  Line_221_to_222_1_mag : Outport  Port=17  VectorParamsAs1DForOutWhenUnconnected=off
  Line_223_to_318_1_mag : Outport  Port=18  VectorParamsAs1DForOutWhenUnconnected=off
  Line_302_to_304_1_mag : Outport  Port=19  VectorParamsAs1DForOutWhenUnconnected=off
  Line_302_to_306_1_mag : Outport  Port=20  VectorParamsAs1DForOutWhenUnconnected=off
  Line_303_to_309_1_mag : Outport  Port=21  VectorParamsAs1DForOutWhenUnconnected=off
  Line_307_to_308_1_mag : Outport  Port=22  VectorParamsAs1DForOutWhenUnconnected=off
  Line_316_to_317_1_mag : Outport  Port=23  VectorParamsAs1DForOutWhenUnconnected=off
  Line_316_to_319_1_mag : Outport  Port=24  VectorParamsAs1DForOutWhenUnconnected=off
  Line_321_to_322_1_mag : Outport  Port=25  VectorParamsAs1DForOutWhenUnconnected=off
  wires:
  Selector/1 -> Line_116_to_117_1_mag/1
  Selector1/1 -> Line_116_to_119_1_mag/1
  Selector2/1 -> Line_121_to_122_1_mag/1
  Selector3/1 -> Line_121_to_325_1_mag/1
  Selector4/1 -> Line_302_to_304_1_mag/1
  Selector5/1 -> Line_302_to_306_1_mag/1
  Selector6/1 -> Line_303_to_309_1_mag/1
  Selector7/1 -> Line_307_to_308_1_mag/1
  Selector13/1 -> Line_102_to_106_1_mag/1
  Selector14/1 -> Line_102_to_104_1_mag/1
  Selector15/1 -> Line_103_to_109_1_mag/1
  Selector16/1 -> Line_107_to_108_1_mag/1
  Selector17/1 -> Line_107_to_203_1_mag/1
  Imag0/1 -> Selector3/1, Selector18/1, Selector19/1, Selector20/1, Selector21/1, Selector22/1, Selector23/1, Selector24/1, Selector26/1, Selector4/1, Selector5/1, Selector6/1, Selector10/1, Selector9/1, Selector8/1, Selector7/1, Selector25/1, Selector2/1, Selector1/1, Selector/1, Selector17/1, Selector16/1, Selector15/1, Selector13/1, Selector14/1
  Selector18/1 -> Line_123_to_217_1_mag/1
  Selector19/1 -> Line_202_to_204_1_mag/1
  Selector20/1 -> Line_202_to_206_1_mag/1
  Selector21/1 -> Line_203_to_209_1_mag/1
  Selector22/1 -> Line_207_to_208_1_mag/1
  Selector23/1 -> Line_216_to_217_1_mag/1
  Selector24/1 -> Line_216_to_219_1_mag/1
  Selector25/1 -> Line_221_to_222_1_mag/1
  Selector26/1 -> Line_223_to_318_1_mag/1
  Selector8/1 -> Line_316_to_317_1_mag/1
  Selector9/1 -> Line_316_to_319_1_mag/1
  Selector10/1 -> Line_321_to_322_1_mag/1

== system System_20220515/sm_master/Subsystem9 ==
  note: Imag1
  Imag1 : Inport
  Terminator : Terminator
  wires:
  Imag1/1 -> Terminator/1

== system System_20220515/sm_master/Timestamp selector ==
  ts_in : Inport
  Demux : Demux  Outputs=8
  Terminator{,1..4} (5 alike) : Terminator
  clock_epoch : rtlab/OpOutput  identifier_use=clock_epoch  identifier_hide=clock_epoch  nb_parents_identifier=0
      settings: SourceProductName=RT-LAB
  clock_ns : rtlab/OpOutput  identifier_use=clock_ns  identifier_hide=clock_ns  nb_parents_identifier=0
      settings: SourceProductName=RT-LAB
  clock_sync : rtlab/OpOutput  identifier_use=clock_sync  identifier_hide=clock_sync  nb_parents_identifier=0
      settings: SourceProductName=RT-LAB
  wires:
  Demux/7 -> clock_epoch/1
  Demux/6 -> clock_ns/1
  Demux/8 -> clock_sync/1
  Demux/1 -> Terminator/1
  Demux/2 -> Terminator1/1
  Demux/3 -> Terminator2/1
  Demux/4 -> Terminator3/1
  Demux/5 -> Terminator4/1
  ts_in/1 -> Demux/1

== system System_20220515/sm_master/bus_va_noise ==
  In1 : Inport
  Add1 : Sum
  MATLAB Function : MATLAB Function  TreatAsAtomicUnit=on
  Random Number : RandomNumber  Variance=ang_variance  Seed=bus_va_seed  SampleTime=Ts
  y : Outport
  wires:
  In1/1 -> Add1/1
  Random Number/1 -> Add1/2
  MATLAB Function/1(y) -> y/1
  Add1/1 -> MATLAB Function/1(u)

== system System_20220515/sm_master/bus_vm_noise ==
  In1 : Inport
  Add1 : Sum
  Random Number : RandomNumber  Variance=mag_variance  Seed=bus_vm_seed  SampleTime=Ts
  Bus_Vm : Outport
  wires:
  In1/1 -> Add1/1
  Random Number/1 -> Add1/2
  Add1/1 -> Bus_Vm/1

== system System_20220515/sm_master/line_iang0_noise ==
  In1 : Inport
  Add1 : Sum
  MATLAB Function : MATLAB Function  TreatAsAtomicUnit=on
  Random Number : RandomNumber  Variance=ang_variance  Seed=line_iang0_seed  SampleTime=Ts
  y : Outport
  wires:
  In1/1 -> Add1/1
  Random Number/1 -> Add1/2
  Add1/1 -> MATLAB Function/1(u)
  MATLAB Function/1(y) -> y/1

== system System_20220515/sm_master/line_iang1_noise ==
  In1 : Inport
  Add1 : Sum
  MATLAB Function : MATLAB Function  TreatAsAtomicUnit=on
  Random Number : RandomNumber  Variance=ang_variance  Seed=line_iang1_seed  SampleTime=Ts
  y : Outport
  wires:
  In1/1 -> Add1/1
  Random Number/1 -> Add1/2
  MATLAB Function/1(y) -> y/1
  Add1/1 -> MATLAB Function/1(u)

== system System_20220515/sm_master/line_imag0_noise ==
  In1 : Inport
  Add1 : Sum
  Random Number : RandomNumber  Variance=mag_variance  Seed=line_imag0_seed  SampleTime=Ts
  Out1 : Outport
  wires:
  In1/1 -> Add1/1
  Random Number/1 -> Add1/2
  Add1/1 -> Out1/1

== system System_20220515/sm_master/line_imag1_noise ==
  In1 : Inport
  Add1 : Sum
  Random Number : RandomNumber  Variance=mag_variance  Seed=line_imag1_seed  SampleTime=Ts
  Out1 : Outport
  wires:
  In1/1 -> Add1/1
  Random Number/1 -> Add1/2
  Add1/1 -> Out1/1

== system System_20220515/sm_master/xf_iang0_noise ==
  In1 : Inport
  Add1 : Sum
  MATLAB Function : MATLAB Function  TreatAsAtomicUnit=on
  Random Number : RandomNumber  Variance=ang_variance  Seed=xf_iang0_seed  SampleTime=Ts
  y : Outport
  wires:
  In1/1 -> Add1/1
  Random Number/1 -> Add1/2
  MATLAB Function/1(y) -> y/1
  Add1/1 -> MATLAB Function/1(u)

== system System_20220515/sm_master/xf_iang1_noise ==
  In1 : Inport
  Add1 : Sum
  MATLAB Function : MATLAB Function  TreatAsAtomicUnit=on
  Random Number : RandomNumber  Variance=ang_variance  Seed=xf_iang1_seed  SampleTime=Ts
  y : Outport
  wires:
  In1/1 -> Add1/1
  Random Number/1 -> Add1/2
  Add1/1 -> MATLAB Function/1(u)
  MATLAB Function/1(y) -> y/1

== system System_20220515/sm_master/xf_imag0_noise ==
  In1 : Inport
  Add1 : Sum
  Random Number : RandomNumber  Variance=mag_variance  Seed=xf_imag0_seed  SampleTime=Ts
  Out1 : Outport
  wires:
  In1/1 -> Add1/1
  Random Number/1 -> Add1/2
  Add1/1 -> Out1/1

== system System_20220515/sm_master/xf_imag1_noise ==
  In1 : Inport
  Add1 : Sum
  Random Number : RandomNumber  Variance=mag_variance  Seed=xf_imag1_seed  SampleTime=Ts
  Out1 : Outport
  wires:
  In1/1 -> Add1/1
  Random Number/1 -> Add1/2
  Add1/1 -> Out1/1

== system System_20220515/sm_master/PMU102_signals/Spoofing attack ==
  note: Modify demux and mux to fit input size.
      | Only modifies the angle measurements.
  Input : Inport
  Add : Sum
  Constant : Constant  Value=en_spoofing_attack.pmu_102
  Demux : Demux  Outputs=8
  Demux1 : Demux
  Multiply : Product
  Mux : Mux  Inputs=8
  Mux1 : Mux
  Ramp : simulink/Sources/Ramp  slope=1*pi()/180  start=spoof_st.pmu_102  InitialOutput=0
  Saturation : Saturate  UpperLimit=spoof_upper_limit  LowerLimit=spoof_lower_limit
  Output : Outport  VectorParamsAs1DForOutWhenUnconnected=off
  wires:
  Multiply/1 -> Add/1
  Saturation/1 -> Multiply/1
  Constant/1 -> Multiply/2
  Ramp/1 -> Saturation/1
  Input/1 -> Demux/1
  Mux/1 -> Output/1
  Demux/1 -> Mux/1
  Demux/3 -> Mux/3
  Demux/5 -> Mux/5
  Demux/7 -> Mux/7
  Demux/8 -> Mux1/4
  Demux/6 -> Mux1/3
  Demux/4 -> Mux1/2
  Demux/2 -> Mux1/1
  Mux1/1 -> Add/2
  Add/1 -> Demux1/1
  Demux1/1 -> Mux/2
  Demux1/2 -> Mux/4
  Demux1/3 -> Mux/6
  Demux1/4 -> Mux/8

== system System_20220515/sm_master/PMU103_signals/Spoofing attack ==
  note: Modify demux and mux to fit input size.
      | Only modifies the angle measurements.
  Input : Inport
  Add : Sum
  Constant : Constant  Value=en_spoofing_attack.pmu_103
  Demux : Demux  Outputs=8
  Demux1 : Demux
  Multiply : Product
  Mux : Mux  Inputs=8
  Mux1 : Mux
  Ramp : simulink/Sources/Ramp  slope=1*pi()/180  start=spoof_st.pmu_103  InitialOutput=0
  Saturation : Saturate  UpperLimit=spoof_upper_limit  LowerLimit=spoof_lower_limit
  Output : Outport  VectorParamsAs1DForOutWhenUnconnected=off
  wires:
  Multiply/1 -> Add/1
  Saturation/1 -> Multiply/1
  Constant/1 -> Multiply/2
  Ramp/1 -> Saturation/1
  Input/1 -> Demux/1
  Mux/1 -> Output/1
  Demux/1 -> Mux/1
  Demux/3 -> Mux/3
  Demux/5 -> Mux/5
  Demux/7 -> Mux/7
  Demux/8 -> Mux1/4
  Demux/6 -> Mux1/3
  Demux/4 -> Mux1/2
  Demux/2 -> Mux1/1
  Mux1/1 -> Add/2
  Add/1 -> Demux1/1
  Demux1/1 -> Mux/2
  Demux1/2 -> Mux/4
  Demux1/3 -> Mux/6
  Demux1/4 -> Mux/8

== system System_20220515/sm_master/PMU107_signals/Spoofing attack ==
  note: Modify demux and mux to fit input size.
      | Only modifies the angle measurements.
  Input : Inport
  Add : Sum
  Constant : Constant  Value=en_spoofing_attack.pmu_107
  Demux : Demux  Outputs=6
  Demux1 : Demux  Outputs=3
  Multiply : Product
  Mux : Mux  Inputs=6
  Mux1 : Mux  Inputs=3
  Ramp : simulink/Sources/Ramp  slope=1*pi()/180  start=spoof_st.pmu_107  InitialOutput=0
  Saturation : Saturate  UpperLimit=spoof_upper_limit  LowerLimit=spoof_lower_limit
  Output : Outport  VectorParamsAs1DForOutWhenUnconnected=off
  wires:
  Multiply/1 -> Add/1
  Saturation/1 -> Multiply/1
  Constant/1 -> Multiply/2
  Ramp/1 -> Saturation/1
  Input/1 -> Demux/1
  Mux/1 -> Output/1
  Demux/1 -> Mux/1
  Demux/3 -> Mux/3
  Demux/5 -> Mux/5
  Demux/6 -> Mux1/3
  Demux/4 -> Mux1/2
  Demux/2 -> Mux1/1
  Mux1/1 -> Add/2
  Add/1 -> Demux1/1
  Demux1/1 -> Mux/2
  Demux1/2 -> Mux/4
  Demux1/3 -> Mux/6

== system System_20220515/sm_master/PMU110_signals/Spoofing attack ==
  note: Modify demux and mux to fit input size.
      | Only modifies the angle measurements.
  Input : Inport
  Add : Sum
  Constant : Constant  Value=en_spoofing_attack.pmu_110
  Demux : Demux  Outputs=12
  Demux1 : Demux  Outputs=6
  Multiply : Product
  Mux : Mux  Inputs=12
  Mux1 : Mux  Inputs=6
  Ramp : simulink/Sources/Ramp  slope=1*pi()/180  start=spoof_st.pmu_110  InitialOutput=0
  Saturation : Saturate  UpperLimit=spoof_upper_limit  LowerLimit=spoof_lower_limit
  Output : Outport  VectorParamsAs1DForOutWhenUnconnected=off
  wires:
  Multiply/1 -> Add/1
  Saturation/1 -> Multiply/1
  Constant/1 -> Multiply/2
  Ramp/1 -> Saturation/1
  Input/1 -> Demux/1
  Mux/1 -> Output/1
  Demux/1 -> Mux/1
  Demux/3 -> Mux/3
  Demux/5 -> Mux/5
  Demux/7 -> Mux/7
  Demux/9 -> Mux/9
  Demux/10 -> Mux1/5
  Demux/8 -> Mux1/4
  Demux/6 -> Mux1/3
  Demux/4 -> Mux1/2
  Demux/2 -> Mux1/1
  Mux1/1 -> Add/2
  Add/1 -> Demux1/1
  Demux1/1 -> Mux/2
  Demux1/2 -> Mux/4
  Demux1/3 -> Mux/6
  Demux1/4 -> Mux/8
  Demux1/5 -> Mux/10
  Demux/11 -> Mux/11
  Demux/12 -> Mux1/6
  Demux1/6 -> Mux/12

== system System_20220515/sm_master/PMU116_signals/Spoofing attack ==
  note: Modify demux and mux to fit input size.
      | Only modifies the angle measurements.
  Input : Inport
  Add : Sum
  Constant : Constant  Value=en_spoofing_attack.pmu_116
  Demux : Demux  Outputs=10
  Demux1 : Demux  Outputs=5
  Multiply : Product
  Mux : Mux  Inputs=10
  Mux1 : Mux  Inputs=5
  Ramp : simulink/Sources/Ramp  slope=1*pi()/180  start=spoof_st.pmu_116  InitialOutput=0
  Saturation : Saturate  UpperLimit=spoof_upper_limit  LowerLimit=spoof_lower_limit
  Output : Outport  VectorParamsAs1DForOutWhenUnconnected=off
  wires:
  Multiply/1 -> Add/1
  Saturation/1 -> Multiply/1
  Constant/1 -> Multiply/2
  Ramp/1 -> Saturation/1
  Input/1 -> Demux/1
  Mux/1 -> Output/1
  Demux/1 -> Mux/1
  Demux/3 -> Mux/3
  Demux/5 -> Mux/5
  Demux/7 -> Mux/7
  Demux/9 -> Mux/9
  Demux/10 -> Mux1/5
  Demux/8 -> Mux1/4
  Demux/6 -> Mux1/3
  Demux/4 -> Mux1/2
  Demux/2 -> Mux1/1
  Mux1/1 -> Add/2
  Add/1 -> Demux1/1
  Demux1/1 -> Mux/2
  Demux1/2 -> Mux/4
  Demux1/3 -> Mux/6
  Demux1/4 -> Mux/8
  Demux1/5 -> Mux/10

== system System_20220515/sm_master/PMU121_signals/Spoofing attack ==
  note: Modify demux and mux to fit input size.
      | Only modifies the angle measurements.
  Input : Inport
  Add : Sum
  Constant : Constant  Value=en_spoofing_attack.pmu_121
  Demux : Demux  Outputs=14
  Demux1 : Demux  Outputs=7
  Multiply : Product
  Mux : Mux  Inputs=14
  Mux1 : Mux  Inputs=7
  Ramp : simulink/Sources/Ramp  slope=1*pi()/180  start=spoof_st.pmu_121  InitialOutput=0
  Saturation : Saturate  UpperLimit=spoof_upper_limit  LowerLimit=spoof_lower_limit
  Output : Outport  VectorParamsAs1DForOutWhenUnconnected=off
  wires:
  Multiply/1 -> Add/1
  Saturation/1 -> Multiply/1
  Constant/1 -> Multiply/2
  Ramp/1 -> Saturation/1
  Input/1 -> Demux/1
  Mux/1 -> Output/1
  Demux/1 -> Mux/1
  Demux/3 -> Mux/3
  Demux/5 -> Mux/5
  Demux/7 -> Mux/7
  Demux/9 -> Mux/9
  Demux/10 -> Mux1/5
  Demux/8 -> Mux1/4
  Demux/6 -> Mux1/3
  Demux/4 -> Mux1/2
  Demux/2 -> Mux1/1
  Mux1/1 -> Add/2
  Add/1 -> Demux1/1
  Demux1/1 -> Mux/2
  Demux1/2 -> Mux/4
  Demux1/3 -> Mux/6
  Demux1/4 -> Mux/8
  Demux1/5 -> Mux/10
  Demux/11 -> Mux/11
  Demux/13 -> Mux/13
  Demux1/6 -> Mux/12
  Demux1/7 -> Mux/14
  Demux/12 -> Mux1/6
  Demux/14 -> Mux1/7

== system System_20220515/sm_master/PMU123_signals/Spoofing attack ==
  note: Modify demux and mux to fit input size.
      | Only modifies the angle measurements.
  Input : Inport
  Add : Sum
  Constant : Constant  Value=en_spoofing_attack.pmu_123
  Demux : Demux  Outputs=12
  Demux1 : Demux  Outputs=6
  Multiply : Product
  Mux : Mux  Inputs=12
  Mux1 : Mux  Inputs=6
  Ramp : simulink/Sources/Ramp  slope=1*pi()/180  start=spoof_st.pmu_123  InitialOutput=0
  Saturation : Saturate  UpperLimit=spoof_upper_limit  LowerLimit=spoof_lower_limit
  Output : Outport  VectorParamsAs1DForOutWhenUnconnected=off
  wires:
  Multiply/1 -> Add/1
  Saturation/1 -> Multiply/1
  Constant/1 -> Multiply/2
  Ramp/1 -> Saturation/1
  Input/1 -> Demux/1
  Mux/1 -> Output/1
  Demux/1 -> Mux/1
  Demux/3 -> Mux/3
  Demux/5 -> Mux/5
  Demux/7 -> Mux/7
  Demux/9 -> Mux/9
  Demux/10 -> Mux1/5
  Demux/8 -> Mux1/4
  Demux/6 -> Mux1/3
  Demux/4 -> Mux1/2
  Demux/2 -> Mux1/1
  Mux1/1 -> Add/2
  Add/1 -> Demux1/1
  Demux1/1 -> Mux/2
  Demux1/2 -> Mux/4
  Demux1/3 -> Mux/6
  Demux1/4 -> Mux/8
  Demux1/5 -> Mux/10
  Demux/11 -> Mux/11
  Demux/12 -> Mux1/6
  Demux1/6 -> Mux/12

== system System_20220515/sm_master/PMU202_signals/Spoofing attack ==
  note: Modify demux and mux to fit input size.
      | Only modifies the angle measurements.
  Input : Inport
  Add : Sum
  Constant : Constant  Value=en_spoofing_attack.pmu_202
  Demux : Demux  Outputs=8
  Demux1 : Demux
  Multiply : Product
  Mux : Mux  Inputs=8
  Mux1 : Mux
  Ramp : simulink/Sources/Ramp  slope=1*pi()/180  start=spoof_st.pmu_202  InitialOutput=0
  Saturation : Saturate  UpperLimit=spoof_upper_limit  LowerLimit=spoof_lower_limit
  Output : Outport  VectorParamsAs1DForOutWhenUnconnected=off
  wires:
  Multiply/1 -> Add/1
  Saturation/1 -> Multiply/1
  Constant/1 -> Multiply/2
  Ramp/1 -> Saturation/1
  Input/1 -> Demux/1
  Mux/1 -> Output/1
  Demux/1 -> Mux/1
  Demux/3 -> Mux/3
  Demux/5 -> Mux/5
  Demux/7 -> Mux/7
  Demux/8 -> Mux1/4
  Demux/6 -> Mux1/3
  Demux/4 -> Mux1/2
  Demux/2 -> Mux1/1
  Mux1/1 -> Add/2
  Add/1 -> Demux1/1
  Demux1/1 -> Mux/2
  Demux1/2 -> Mux/4
  Demux1/3 -> Mux/6
  Demux1/4 -> Mux/8

== system System_20220515/sm_master/PMU203_signals/Spoofing attack ==
  note: Modify demux and mux to fit input size.
      | Only modifies the angle measurements.
  Input : Inport
  Add : Sum
  Constant : Constant  Value=en_spoofing_attack.pmu_203
  Demux : Demux  Outputs=10
  Demux1 : Demux  Outputs=5
  Multiply : Product
  Mux : Mux  Inputs=10
  Mux1 : Mux  Inputs=5
  Ramp : simulink/Sources/Ramp  slope=1*pi()/180  start=spoof_st.pmu_203  InitialOutput=0
  Saturation : Saturate  UpperLimit=spoof_upper_limit  LowerLimit=spoof_lower_limit
  Output : Outport  VectorParamsAs1DForOutWhenUnconnected=off
  wires:
  Multiply/1 -> Add/1
  Saturation/1 -> Multiply/1
  Constant/1 -> Multiply/2
  Ramp/1 -> Saturation/1
  Input/1 -> Demux/1
  Mux/1 -> Output/1
  Demux/1 -> Mux/1
  Demux/3 -> Mux/3
  Demux/5 -> Mux/5
  Demux/7 -> Mux/7
  Demux/9 -> Mux/9
  Demux/10 -> Mux1/5
  Demux/8 -> Mux1/4
  Demux/6 -> Mux1/3
  Demux/4 -> Mux1/2
  Demux/2 -> Mux1/1
  Mux1/1 -> Add/2
  Add/1 -> Demux1/1
  Demux1/1 -> Mux/2
  Demux1/2 -> Mux/4
  Demux1/3 -> Mux/6
  Demux1/4 -> Mux/8
  Demux1/5 -> Mux/10
